simulink model "exercise1_sl"  (R2019b)
settings: Solver=FixedStepAuto  StartTime=0.0  StopTime=10.0  FixedStep=1e-3  RelTol=1e-3  EnableMultiTasking=on
settings Model: ExtModeTrigMode=oneshot  ExtModeArmWhenConnect=off  Creator=lucam  LastModifiedBy=lucam
settings DataIOCC: SaveFormat=Array  SignalLoggingSaveFormat=ModelDataLogs  ReturnWorkspaceOutputs=off
settings OptimizationCC: BlockReduction=off  BooleanDataType=off
settings DebuggingCC: SaveWithParameterizedLinksMsg=none  UnderspecifiedInitializationDetection=Classic  MergeDetectMultiDrivingBlocksExec=none  SignalResolutionControl=TryResolveAllWithWarning  MultiTaskDSMMsg=warning  MultiTaskCondExecSysMsg=none  ArithmeticOperatorsInVariantConditions=warning
settings HardwareCC: TargetUnknown=on
settings ModelReferenceCC: PropagateSignalLabelsOutOfModel=off
settings SFSimCC: SimUseLocalCustomCode=off  CustomCodeUndefinedFunction=UseInterfaceOnly
settings RTWCC: RTWUseLocalCustomCode=off
settings GRTTargetCC: TargetLangStandard=C89/C90 (ANSI)  CombineOutputUpdateFcns=off  GRTInterface=on

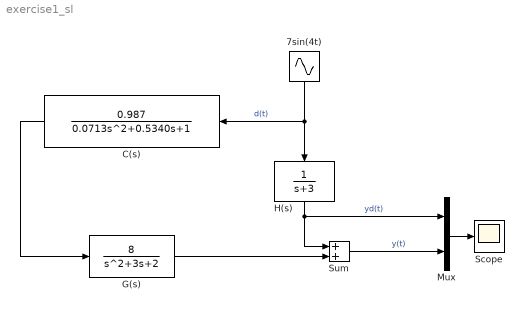
== system exercise1_sl ==
  7sin(4t) : Sin  Amplitude=7  Frequency=4  SampleTime=0
  C(s) : TransferFcn  Numerator=0.987  Denominator=[0.0713 0.5340 1]
  G(s) : TransferFcn  Numerator=8  Denominator=[1 3 2]
  H(s) : TransferFcn  Denominator=[1 3]
  Mux : Mux  Inputs=2
  Scope : Scope
  Sum : Sum  SaturateOnIntegerOverflow=on  InputSameDT=on  OutDataTypeStr=Inherit: Same as first input
  wires:
  7sin(4t)/1 -> H(s)/1, C(s)/1  "d(t)"
  C(s)/1 -> G(s)/1
  G(s)/1 -> Sum/2
  Mux/1 -> Scope/1
  H(s)/1 -> Sum/1, Mux/1  "yd(t)"
  Sum/1 -> Mux/2  "y(t)"
